simulink model "Problem2"  (R2021a)
settings: Solver=VariableStepAuto  StartTime=0.0  StopTime=10.0  RelTol=1e-3
model workspace (MAT data in the model file):
  K = 0.01
  b = 50
  k = 0.02
  k1 = 50
  k2 = 20
settings Model: ParameterArgumentNames=K,b,k,k1,k2  OrderedModelArguments=off  Creator=Nida  LastModifiedBy=Nida

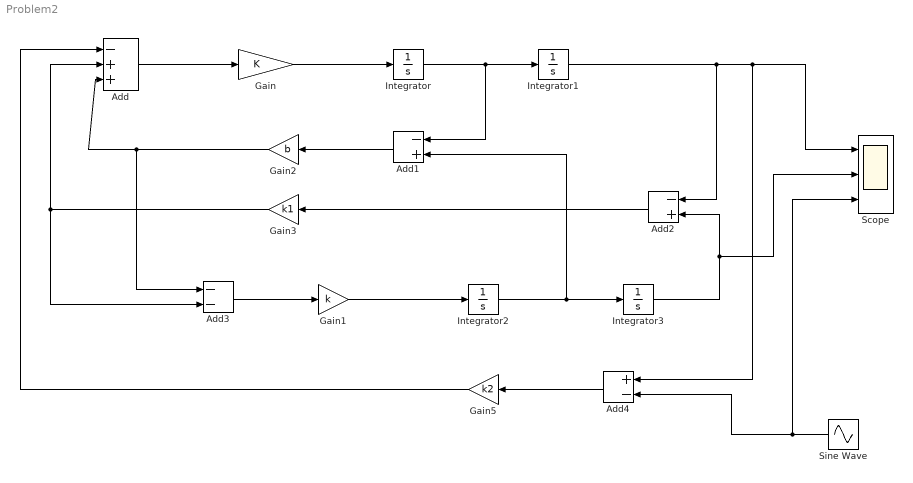
== system Problem2 ==
  Add : Sum  Inputs=-++
  Add1 : Sum  Inputs=-+
  Add2 : Sum  Inputs=-+
  Add3 : Sum  Inputs=--
  Add4 : Sum  Inputs=+-
  Gain : Gain  Gain=K
  Gain1 : Gain  Gain=k
  Gain2 : Gain  Gain=b
  Gain3 : Gain  Gain=k1
  Gain5 : Gain  Gain=k2
  Integrator{,1..3} (4 alike) : Integrator
  Scope : Scope  NumInputPorts=3
  Sine Wave : Sin  SampleTime=0
  wires:
  Add/1 -> Gain/1
  Gain/1 -> Integrator/1
  Integrator/1 -> Add1/1, Integrator1/1
  Add1/1 -> Gain2/1
  Add2/1 -> Gain3/1
  Integrator1/1 -> Add2/1, Add4/1, Scope/1
  Gain1/1 -> Integrator2/1
  Integrator2/1 -> Add1/2, Integrator3/1
  Gain5/1 -> Add/1
  Add3/1 -> Gain1/1
  Gain3/1 -> Add3/2, Add/2
  Gain2/1 -> Add3/1, Add/3
  Add4/1 -> Gain5/1
  Sine Wave/1 -> Scope/3, Add4/2
  Integrator3/1 -> Add2/2, Scope/2
